simulink model "step5_setup_obsservor_test1"  (R2021b)
settings: Solver=FixedStepAuto  StartTime=0.0  StopTime=RunTime  FixedStep=time_step  RelTol=1e-3
values from neighbouring files (symbols this model uses):
  A = double(A)    [step4_0_linearize_operating_point.m]    (also in step4_linearized_system.mat = [0 -1.79155728996 0 111.114105003 0 1 -687.855245355 0 1440.)
  adingain = [adin_gain 1 1 1 1 1]    [hwinit.m]
  adinoffs = [-adin_offs 0 0 0 0 0]    [hwinit.m]
  B = double(B)    [step4_0_linearize_operating_point.m]    (also in step4_linearized_system.mat = [0 0 0 0 2553.84140127])
  C = [1 0 0 0 0 ... (first row only)    [step4_0_linearize_operating_point.m]    (also in step4_linearized_system.mat = [1  0  0  0  0; 0  0  1  0  0])
  daoutgain = 1*[-6]    [hwinit.m]
  daoutoffs = [0.00]    [hwinit.m]
  g1 = (m_1 * c_1_0 + m_2 * l_1) * g    [compare_ourmodel_with_others.m]    (also in step4_0_linearize_operating_point.m = (m1 * c1 + m2 * l1) * g; step6_1_controller_feedback.m = (m1 * c1 + m2 * l1) * g)
  g2 = m_2 * c_2_0 * g    [compare_ourmodel_with_others.m]    (also in step4_0_linearize_operating_point.m = m2 * c2 * g; step6_1_controller_feedback.m = m2 * c2 * g)
  h = 0.001    [hwinit.m]    (also in init_fugi.m = fugiboard('Open', 'pendulum1'); rotpentest.m = fugiboard('Open', 'pendulum1'))
  Ke = [-1014.32161654  -177.47537744; 695281.543064  120402.504185; 2277.4140173  444.622636664; -1453617.5345  -250792.704056; -2689.50349386  -1194.73697046]    [step5_observor.mat]
  P1 = m_1 * c_1_0 * c_1_0 + m_2 * l_1 * l_1 + I_1_0    [compare_ourmodel_with_others.m]    (also in step4_0_linearize_operating_point.m = m1 * c1 * c1 + m2 * l1 * l1 + I1; step6_1_controller_feedback.m = m1 * c1 * c1 + m2 * l1 * l1 + I1)
  P2 = m_2 * c_2_0 * c_2_0 + I_2_0    [compare_ourmodel_with_others.m]    (also in step4_0_linearize_operating_point.m = m2 * c2 * c2 + I2; step6_1_controller_feedback.m = m2 * c2 * c2 + I2)
  P3 = m_2 * l_1 * c_2_0    [compare_ourmodel_with_others.m]    (also in step4_0_linearize_operating_point.m = m2 * l1 * c2; step6_1_controller_feedback.m = m2 * l1 * c2)
  params = [9.81, 0.1, 0.1, 0.125, 0.0487, -0.0286, 0.0624, 0.0169, 6.81e-5, 6.9742, 2.89e-05, 46.1069, 0.0308]    [compare_ourmodel_with_others.m]    (also in costfun.m = x; step2_whitebox_pend.m = x; step4_linearized_system.mat = [9.81 0.1 0.1 0.125 0.046955 -0.032 0.04609 0.0088 9.8e-05 6)
  theta_1_0 = pi    (= 3.14159265359)    [hwinit.m]    (also in step4_0_linearize_operating_point.m = 0; step6_1_controller_feedback.m = 0)
  theta_2_0 = 0    [hwinit.m]    (also in step4_0_linearize_operating_point.m; step6_1_controller_feedback.m)
  x_op_relative = [0; 0; 0; 0; 0]    [step6_1_controller_feedback.m]
settings Model: LastModifiedBy=lyitingli
settings OptimizationCC: BlockReduction=off  BooleanDataType=off
settings DebuggingCC: SaveWithParameterizedLinksMsg=none  UnderspecifiedInitializationDetection=Classic  MergeDetectMultiDrivingBlocksExec=none  SignalResolutionControl=TryResolveAllWithWarning
settings HardwareCC: TargetUnknown=on
settings ModelReferenceCC: PropagateSignalLabelsOutOfModel=off

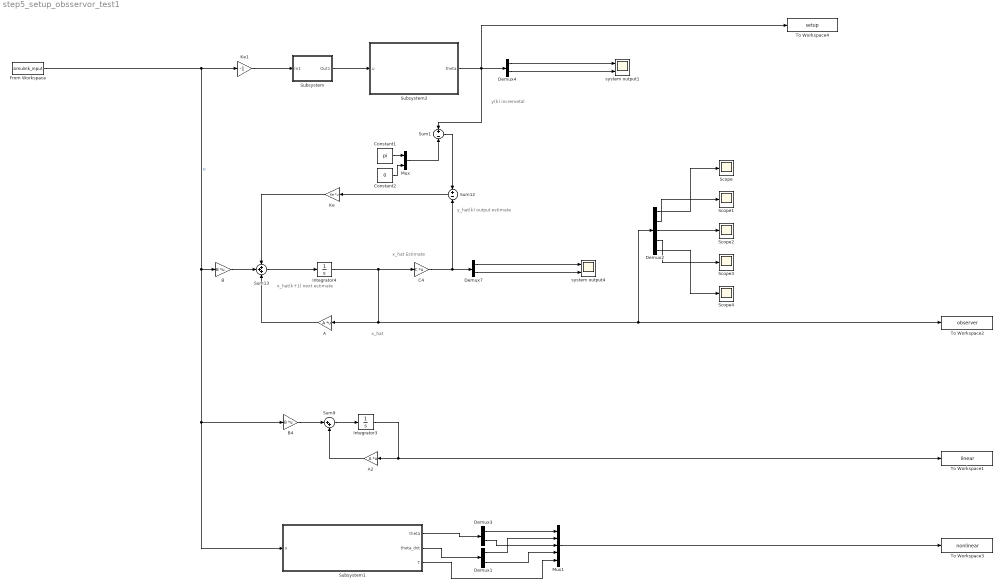
== system step5_setup_obsservor_test1 ==
  note: y_hat(k)
      | output estimate
  note: x_hat(k+1)
      | next estimate
  note: y(k)
      | incremetal
  note: x_hat
      | Estimate
  note: x_hat
  A : Gain  Gain=A  Multiplication=Matrix(K*u) (u vector)
  A2 : Gain  Gain=A  Multiplication=Matrix(K*u) (u vector)
  B : Gain  Gain=B  Multiplication=Matrix(K*u)
  B4 : Gain  Gain=B  Multiplication=Matrix(K*u)
  C4 : Gain  Gain=C  Multiplication=Matrix(K*u) (u vector)
  Constant1 : Constant  Value=pi  SampleTime=-1
  Constant2 : Constant  Value=0  SampleTime=-1
  Demux{1,3..4,7} (4 alike) : Demux  Outputs=2
  Demux2 : Demux  Outputs=5
  From Workspace : FromWorkspace  SampleTime=-1
  Integrator3 : Integrator  InitialCondition=x_op_relative
  Integrator4 : Integrator  InitialCondition=[0; 0; 0; 0; 0]
  Ke : Gain  Gain=Ke  Multiplication=Matrix(K*u) (u vector)
  Ke1 : Gain  Gain=-1
  Mux : Mux  Inputs=2
  Mux1 : Mux  Inputs=5
  Scope{,1..4} (5 alike) : Scope
  Subsystem : Subsystem
      mask Display: disp('Rotational\nPendulum')
  Subsystem1 : Subsystem
  Subsystem2 : Subsystem
  Sum1 : Sum  Inputs=+|-
  Sum12 : Sum  Inputs=+|-
  Sum13 : Sum  Inputs=+++
  Sum9 : Sum  Inputs=|++
  To Workspace1 : ToWorkspace  VariableName=linear  SampleTime=0.001
  To Workspace2 : ToWorkspace  VariableName=observer  SampleTime=0.001
  To Workspace3 : ToWorkspace  VariableName=nonlinear  SampleTime=0.001
  To Workspace4 : ToWorkspace  VariableName=setup  SampleTime=0.001
  system output1 : Scope  NumInputPorts=2
  system output4 : Scope  NumInputPorts=2
  wires:
  Demux7/1 -> system output4/1
  Ke/1 -> Sum13/1
  A/1 -> Sum13/3
  Demux7/2 -> system output4/2
  Sum13/1 -> Integrator4/1
  B/1 -> Sum13/2
  Sum1/1 -> Sum12/1
  Constant1/1 -> Mux/1
  Constant2/1 -> Mux/2
  Mux/1 -> Sum1/2
  Subsystem/1(Out1) -> Subsystem2/1(u)
  Sum12/1 -> Ke/1
  C4/1 -> Sum12/2, Demux7/1
  Integrator4/1 -> Demux2/1, To Workspace2/1, A/1, C4/1
  B4/1 -> Sum9/1
  Sum9/1 -> Integrator3/1
  A2/1 -> Sum9/2
  Integrator3/1 -> A2/1, To Workspace1/1
  From Workspace/1 -> Subsystem1/1(u), B4/1, B/1, Ke1/1  "u"
  Subsystem1/1(theta) -> Demux3/1
  Subsystem1/2(theta_dot) -> Demux1/1
  Demux3/1 -> Mux1/1
  Demux3/2 -> Mux1/3
  Demux1/1 -> Mux1/2
  Demux1/2 -> Mux1/4
  Mux1/1 -> To Workspace3/1
  Subsystem1/3(T) -> Mux1/5
  Demux2/1 -> Scope/1
  Demux2/2 -> Scope1/1
  Demux2/3 -> Scope2/1
  Demux2/4 -> Scope3/1
  Demux2/5 -> Scope4/1
  Ke1/1 -> Subsystem/1(In1)
  Demux4/2 -> system output1/2
  Demux4/1 -> system output1/1
  Subsystem2/1(theta) -> To Workspace4/1, Demux4/1, Sum1/1

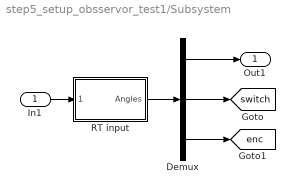
== system step5_setup_obsservor_test1/Subsystem ==
  In1 : Inport
  Demux : Demux  Outputs=[2 4 1]
  RT input : Subsystem  mask{Ts=h, channels=[6 7]}
      mask prompts: Ts "Sample time [s]:"; channels "Channels to read (e.g., [6 7])"
      mask init:
      | hwinit;
      | 
      | % initialize FPGA
      | fugihandle = fugiboard('Open', 'Pendulum1');
      | fugihandle.WatchdogTimeout = 0.5;
      | fugiboard('SetParams', fugihandle);
      | fugiboard('Write', fugihandle, 0, 0, 0, 0);  % dummy write to sync interface board
      | fugiboard('Write', fugihandle, 5, 1, 0, 0);  % reset position, activate relay
      | data = fugiboard('Read', fugihandle);        % get version info from FPGA
      | % model = bitshift(data(1), -5); 
      | % version = bitand(data(1), 31);
      | % disp(sprintf('FPGA setup %d, version %d', model, version)); % for the B&P it should say 1 1, or else there is a problem
      | fugiboard('Write', fugihandle, 0, 1, 0, 0);  % end reset
      | pause(0.1);                         % give relay some time to respond
      mask Display: disp('Rotational\nPendulum')
  Out1 : Outport
  tag scope: enc=global, switch=global
  wires:
  RT input/1(Angles) -> Demux/1
  Demux/1 -> Out1/1
  Demux/2 -> [switch]
  Demux/3 -> [enc]
  In1/1 -> RT input/1(Motors)

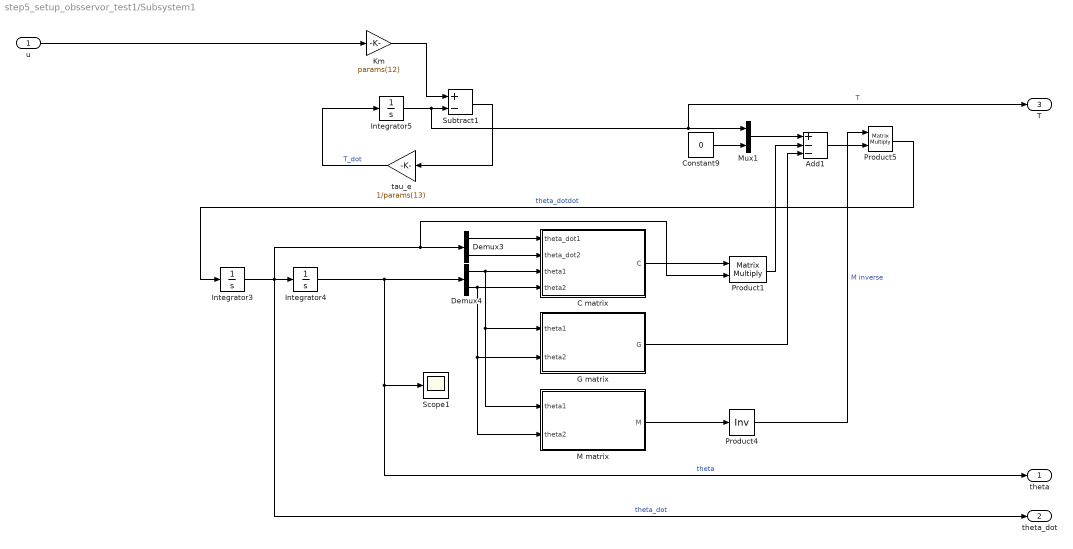
== system step5_setup_obsservor_test1/Subsystem1 ==
  u : Inport
  Add1 : Sum  Inputs=+--
  C matrix : MATLAB Function  TreatAsAtomicUnit=on
  Constant9 : Constant  Value=0
  Demux3 : Demux  Outputs=2
  Demux4 : Demux  Outputs=2
  G matrix : MATLAB Function  TreatAsAtomicUnit=on
  Integrator3 : Integrator
  Integrator4 : Integrator  InitialCondition=[theta_1_0 theta_2_0]
  Integrator5 : Integrator
  Km : Gain  Gain=params(12)
  M matrix : MATLAB Function  TreatAsAtomicUnit=on
  Mux1 : Mux  Inputs=2
  Product1 : Product  Inputs=**  Multiplication=Matrix(*)
  Product4 : Product  Inputs=/  Multiplication=Matrix(*)
  Product5 : Product  Inputs=**  Multiplication=Matrix(*)
  Scope1 : Scope
  Subtract1 : Sum  Inputs=+-
  tau_e : Gain  Gain=1/params(13)
  theta : Outport
  theta_dot : Outport  Port=2
  T : Outport  Port=3
  wires:
  Demux4/1 -> M matrix/1(theta1), G matrix/1(theta1), C matrix/3(theta1)
  tau_e/1 -> Integrator5/1  "T_dot"
  Constant9/1 -> Mux1/2
  Demux3/1 -> C matrix/1(theta_dot1)
  Add1/1 -> Product5/2
  Subtract1/1 -> tau_e/1
  G matrix/1(G) -> Add1/3
  Integrator3/1 -> theta_dot/1, Product1/2, Demux3/1, Integrator4/1  "theta_dot"
  C matrix/1(C) -> Product1/1
  Mux1/1 -> Add1/1
  Integrator5/1 -> T/1, Mux1/1, Subtract1/2  "T"
  u/1 -> Km/1
  Product5/1 -> Integrator3/1  "theta_dotdot"
  Demux3/2 -> C matrix/2(theta_dot2)
  Integrator4/1 -> Demux4/1, theta/1, Scope1/1  "theta"
  M matrix/1(M) -> Product4/1
  Demux4/2 -> M matrix/2(theta2), G matrix/2(theta2), C matrix/4(theta2)
  Product4/1 -> Product5/1  "M inverse"
  Product1/1 -> Add1/2
  Km/1 -> Subtract1/1

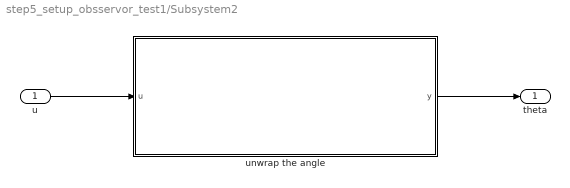
== system step5_setup_obsservor_test1/Subsystem2 ==
  u : Inport
  unwrap the angle : MATLAB Function  TreatAsAtomicUnit=on
  theta : Outport
  wires:
  u/1 -> unwrap the angle/1(u)
  unwrap the angle/1(y) -> theta/1

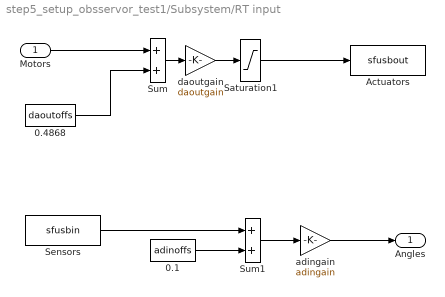
== system step5_setup_obsservor_test1/Subsystem/RT input ==
  Motors : Inport
  0.1 : Constant  Value=adinoffs
  0.4868 : Constant  Value=daoutoffs
  Actuators : S-Function  FunctionName=sfusbout  Parameters=Ts, fugihandle  SFunctionDeploymentMode=off  EnableBusSupport=off
  Saturation1 : Saturate  UpperLimit=10  LowerLimit=-10
  Sensors : S-Function  FunctionName=sfusbin  Parameters=Ts, fugihandle, channels  SFunctionDeploymentMode=off  EnableBusSupport=off
  Sum : Sum  InputSameDT=on  SaturateOnIntegerOverflow=on  OutDataTypeStr=Inherit: Same as first input
  Sum1 : Sum  InputSameDT=on  SaturateOnIntegerOverflow=on  OutDataTypeStr=Inherit: Same as first input
  adingain : Gain  Gain=adingain  SaturateOnIntegerOverflow=on  OutDataTypeStr=Inherit: Same as input  ParamDataTypeStr=Inherit: Same as input
  daoutgain : Gain  Gain=daoutgain  SaturateOnIntegerOverflow=on  OutDataTypeStr=Inherit: Same as input  ParamDataTypeStr=Inherit: Same as input
  Angles : Outport
  wires:
  Sum/1 -> daoutgain/1
  0.4868/1 -> Sum/2
  Motors/1 -> Sum/1
  Sum1/1 -> adingain/1
  0.1/1 -> Sum1/2
  adingain/1 -> Angles/1
  Saturation1/1 -> Actuators/1
  daoutgain/1 -> Saturation1/1
  Sensors/1 -> Sum1/1

== matlab function step5_setup_obsservor_test1/Subsystem1/C matrix ==
  data: theta_dot1 input; theta_dot2 input; theta1 input; theta2 input; C output; params parameter; P3 parameter
function C = C(theta_dot1, theta_dot2, theta1, theta2, params, P3)
c00 = params(10) - P3 * theta_dot2 * sin(theta2);
c01 = -P3 * (theta_dot1 + theta_dot2) * sin(theta2);
c10 = P3 * theta_dot1 * sin(theta2);
c11 = params(11);

C = [c00 c01;
     c10 c11];

== matlab function step5_setup_obsservor_test1/Subsystem1/G matrix ==
  data: theta1 input; theta2 input; G output; g1 parameter; g2 parameter
function G = G(theta1, theta2, g1, g2)
G00 = -g1 * sin(theta1) - g2 * sin(theta1 + theta2);
G01 = -g2 * sin(theta1 + theta2);

G = [G00 G01];

== matlab function step5_setup_obsservor_test1/Subsystem1/M matrix ==
  data: theta1 input; theta2 input; M output; P1 parameter; P2 parameter; P3 parameter
function M = fcn(theta1, theta2, P1, P2, P3)
M00 = P1 + P2 + 2 * P3 * cos(theta2);
M01 = P2 + P3 * cos(theta2);
M10 = M01;
M11 = P2;

M = [M00 M01;
     M10 M11];

== matlab function step5_setup_obsservor_test1/Subsystem2/unwrap the angle ==
  settings: updateMethod=DISCRETE  sampleTime=0.001
  data: u input size=2; y output size=2
function y = unwrap_angle(u)

y = unwrap(u);
% y = u;
